simulink model "float2uint8_code_decode_TEST"  (R2018b)
settings: Solver=FixedStepAuto  StartTime=0.0  StopTime=10.0  RelTol=1e-3
model workspace (MAT data in the model file):
  precision = 4
libraries: hdlsllib x3
settings Model: Creator=Diego  LastModifiedBy=Diego

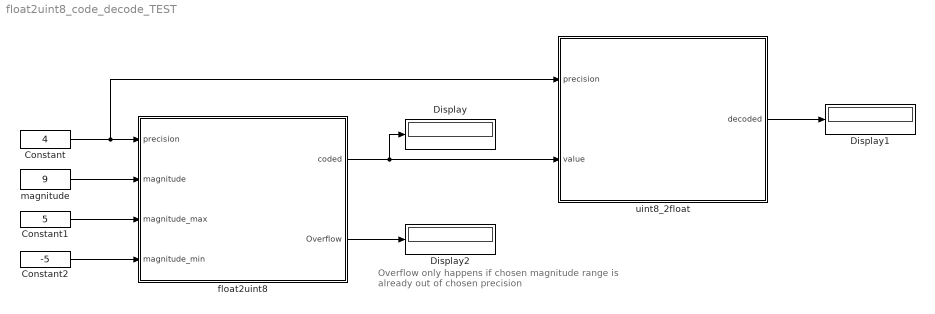
== system float2uint8_code_decode_TEST ==
  note: Overflow only happens if chosen magnitude range
      | is already out of chosen precision
  Constant : Constant  Value=4
  Constant1 : Constant  Value=5
  Constant2 : Constant  Value=-5
  Display : Display
  Display1 : Display
  Display2 : Display
  float2uint8 : Subsystem
  magnitude : Constant  Value=9
  uint8_2float : Subsystem
  wires:
  float2uint8/1(coded) -> Display/1, uint8_2float/2(value)
  magnitude/1 -> float2uint8/2(magnitude)
  Constant/1 -> float2uint8/1(precision), uint8_2float/1(precision)
  uint8_2float/1(decoded) -> Display1/1
  float2uint8/2(Overflow) -> Display2/1
  Constant1/1 -> float2uint8/3(magnitude_max)
  Constant2/1 -> float2uint8/4(magnitude_min)

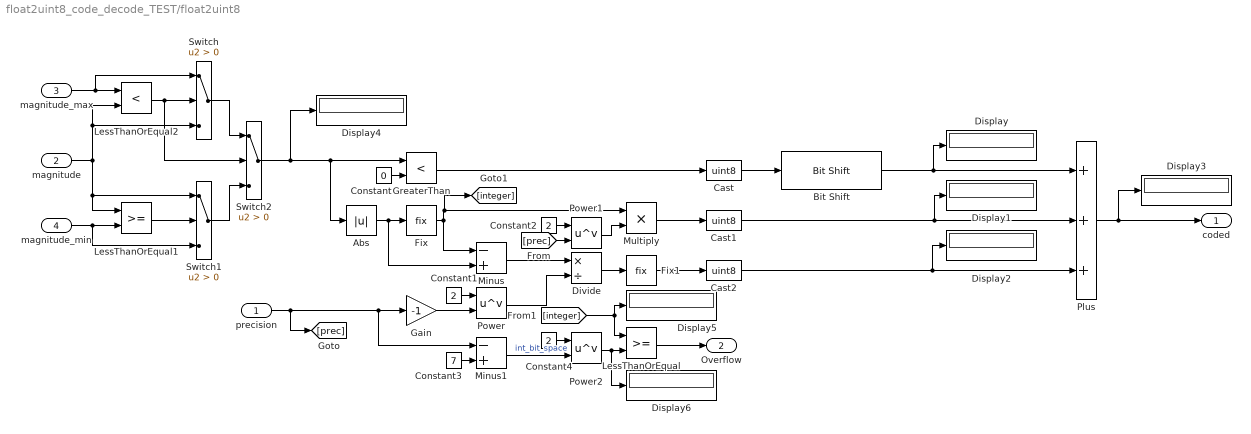
== system float2uint8_code_decode_TEST/float2uint8 ==
  precision : Inport
  magnitude : Inport  Port=2
  magnitude_max : Inport  Port=3
  magnitude_min : Inport  Port=4
  Abs : Abs
  Bit Shift : hdlsllib/Logic and Bit Operations/Bit Shift  mode=Shift Left Logical  N=7
      settings: SourceProductName=HDL Coder  SourceProductBaseCode=HD
  Cast : DataTypeConversion  OutDataTypeStr=uint8
  Cast1 : DataTypeConversion  OutDataTypeStr=uint8
  Cast2 : DataTypeConversion  OutDataTypeStr=uint8
  Constant : Constant  Value=0
  Constant1 : Constant  Value=2
  Constant2 : Constant  Value=2
  Constant3 : Constant  Value=7
  Constant4 : Constant  Value=2
  Display{,1..6} (7 alike) : Display
  Divide : Product  Inputs=*/
  Fix : Rounding  Priority=3  Operator=fix
  Fix1 : Rounding  Priority=6  Operator=fix
  Gain : Gain  Gain=-1
  GreaterThan : RelationalOperator  Priority=2  Operator=<  OutDataTypeStr=boolean  RndMeth=Simplest
  LessThanOrEqual : RelationalOperator  OutDataTypeStr=boolean  RndMeth=Simplest
  LessThanOrEqual1 : RelationalOperator  OutDataTypeStr=boolean  RndMeth=Simplest
  LessThanOrEqual2 : RelationalOperator  Operator=<  OutDataTypeStr=boolean  RndMeth=Simplest
  Minus : Sum  Priority=4  Inputs=-+
  Minus1 : Sum  Priority=4  Inputs=-+
  Multiply : Product
  Plus : Sum  Priority=10  Inputs=+++
  Power : Math  Priority=5  Operator=pow  SaturateOnIntegerOverflow=on
  Power1 : Math  Priority=5  Operator=pow  SaturateOnIntegerOverflow=on
  Power2 : Math  Priority=5  Operator=pow  SaturateOnIntegerOverflow=on
  Switch : Switch  Criteria=u2 > Threshold
  Switch1 : Switch  Criteria=u2 > Threshold
  Switch2 : Switch  Criteria=u2 > Threshold
  coded : Outport
  Overflow : Outport  Port=2
  wires:
  Constant/1 -> GreaterThan/2
  Switch2/1 -> Display4/1, Abs/1, GreaterThan/1
  Abs/1 -> Minus/2, Fix/1
  GreaterThan/1 -> Cast/1
  Fix/1 -> [integer], Multiply/1, Minus/1
  Minus/1 -> Divide/1
  Cast/1 -> Bit Shift/1
  Bit Shift/1 -> Display/1, Plus/1
  Cast1/1 -> Display1/1, Plus/2
  Constant1/1 -> Power/1
  Gain/1 -> Power/2
  Power/1 -> Divide/2
  Divide/1 -> Fix1/1
  Fix1/1 -> Cast2/1
  Cast2/1 -> Display2/1, Plus/3
  Constant2/1 -> Power1/1
  Power1/1 -> Multiply/2
  precision/1 -> [prec], Minus1/1, Gain/1
  Multiply/1 -> Cast1/1
  [prec] -> Power1/2
  Constant3/1 -> Minus1/2
  Minus1/1 -> Power2/2  "int_bit_space"
  Constant4/1 -> Power2/1
  Power2/1 -> Display6/1, LessThanOrEqual/2
  LessThanOrEqual/1 -> Overflow/1
  Plus/1 -> coded/1, Display3/1
  magnitude/1 -> LessThanOrEqual1/1, Switch1/1, LessThanOrEqual2/2, Switch/3
  magnitude_min/1 -> LessThanOrEqual1/2, Switch1/3
  magnitude_max/1 -> Switch/1, LessThanOrEqual2/1
  LessThanOrEqual2/1 -> Switch2/2, Switch/2
  LessThanOrEqual1/1 -> Switch1/2
  Switch/1 -> Switch2/1
  Switch1/1 -> Switch2/3
  [integer] -> Display5/1, LessThanOrEqual/1

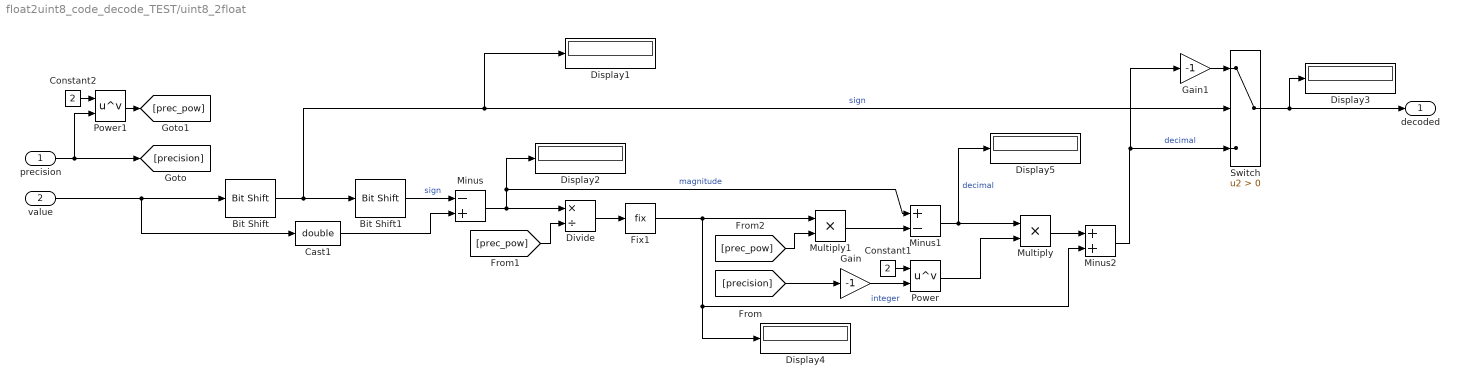
== system float2uint8_code_decode_TEST/uint8_2float ==
  precision : Inport
  value : Inport  Port=2
  Bit Shift : hdlsllib/Logic and Bit Operations/Bit Shift  mode=Shift Right Logical  N=7
      settings: SourceProductName=HDL Coder  SourceProductBaseCode=HD
  Bit Shift1 : hdlsllib/Logic and Bit Operations/Bit Shift  mode=Shift Left Logical  N=7
      settings: SourceProductName=HDL Coder  SourceProductBaseCode=HD
  Cast1 : DataTypeConversion  OutDataTypeStr=double
  Constant1 : Constant  Value=2
  Constant2 : Constant  Value=2
  Display{1..5} (5 alike) : Display
  Divide : Product  Inputs=*/
  Fix1 : Rounding  Operator=fix
  Gain : Gain  Gain=-1
  Gain1 : Gain  Gain=-1
  Minus : Sum  Inputs=-+
  Minus1 : Sum  Inputs=+-
  Minus2 : Sum
  Multiply : Product
  Multiply1 : Product
  Power : Math  Priority=5  Operator=pow  SaturateOnIntegerOverflow=on
  Power1 : Math  Priority=5  Operator=pow  SaturateOnIntegerOverflow=on
  Switch : Switch  Criteria=u2 > Threshold
  decoded : Outport
  wires:
  Bit Shift/1 -> Bit Shift1/1, Switch/2, Display1/1  "sign"
  value/1 -> Cast1/1, Bit Shift/1
  Minus/1 -> Divide/1, Display2/1, Minus1/1  "magnitude"
  Fix1/1 -> Minus2/2, Display4/1, Multiply1/1  "integer"
  Multiply1/1 -> Minus1/2
  Minus1/1 -> Display5/1, Multiply/1  "decimal"
  Constant1/1 -> Power/1
  Gain/1 -> Power/2
  Power/1 -> Multiply/2
  [precision] -> Gain/1
  Multiply/1 -> Minus2/1
  Minus2/1 -> Gain1/1, Switch/3  "decimal"
  Gain1/1 -> Switch/1
  Switch/1 -> Display3/1, decoded/1
  Divide/1 -> Fix1/1
  Cast1/1 -> Minus/2
  precision/1 -> Power1/2, [precision]
  Constant2/1 -> Power1/1
  Power1/1 -> [prec_pow]
  [prec_pow] -> Divide/2
  [prec_pow] -> Multiply1/2
  Bit Shift1/1 -> Minus/1  "sign"
